simulink model "bh_3d_pend_sim_compare"  (R2017a)
settings: Solver=ode45  StartTime=0.0  StopTime=11  RelTol=1e-5  EnableMultiTasking=on
undefined symbols (not defined in the file or in its folder): DOT_Phi_Theta_Psi, DOT_XYZ, g, Hx, Hy, Hz, Lx, Ly, Lz, M_cart, m_pend, Phi_Theta_Psi, q0_ang_deg, q0_dot_and_deg, X, XYZ, Y, Z
libraries: nesl_utility x14, sm_lib x9, simulink_extras x5
settings Model: Creator=bhorton  LastModifiedBy=bhorton
settings SolverCC: ZeroCrossAlgorithm=Adaptive
settings DataIOCC: LimitDataPoints=on
settings OptimizationCC: LifeSpan=inf
settings DebuggingCC: AllowSymbolicDim=off  SFUnexpectedBacktrackingDiag=warning  SFNoUnconditionalDefaultTransitionDiag=warning  SFExecutionAtInitializationDiag=none
settings GRTTargetCC: TargetLangStandard=C89/C90 (ANSI)  GeneratePreprocessorConditionals=Disable all
settings ConfigComp: CovMetricSettings=dw  CovHtmlReporting=on  CovSaveCumulativeToWorkspaceVar=on  CovSaveSingleToWorkspaceVar=on  CovExternalEMLEnable=off  CovSFcnEnable=off
settings SimscapeCC: SimscapeLogType=all  SimscapeLogDataHistory=10000
settings ConfigurationSet: Description=SimMechanics 2G

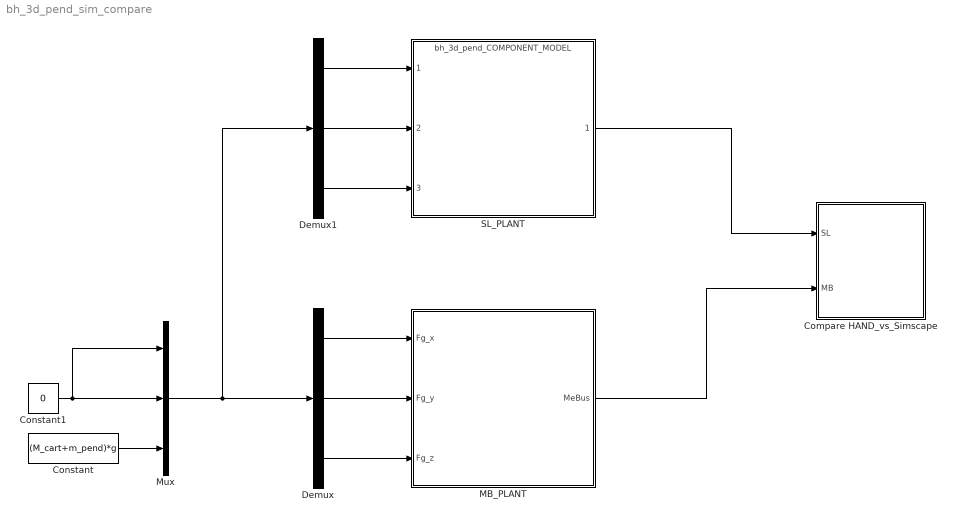
== system bh_3d_pend_sim_compare ==
  Compare HAND_vs_Simscape : Subsystem
  Constant : Constant  Value=(M_cart+m_pend)*g
  Constant1 : Constant  Value=0
  Demux : Demux  Outputs=3
  Demux1 : Demux  Outputs=3
  MB_PLANT : Subsystem
  Mux : Mux  Inputs=3
  SL_PLANT : ModelReference  ModelNameDialog=bh_3d_pend_COMPONENT_MODEL.slx  SimulationMode=Normal  ModelReferenceVersion=1.15
  wires:
  Constant/1 -> Mux/3
  Constant1/1 -> Mux/1, Mux/2
  Demux/1 -> MB_PLANT/1(Fg_x)
  Demux/3 -> MB_PLANT/3(Fg_z)
  Demux/2 -> MB_PLANT/2(Fg_y)
  Mux/1 -> Demux1/1, Demux/1
  Demux1/1 -> SL_PLANT/1
  Demux1/2 -> SL_PLANT/2
  Demux1/3 -> SL_PLANT/3
  SL_PLANT/1 -> Compare HAND_vs_Simscape/1(SL)
  MB_PLANT/1(MeBus) -> Compare HAND_vs_Simscape/2(MB)

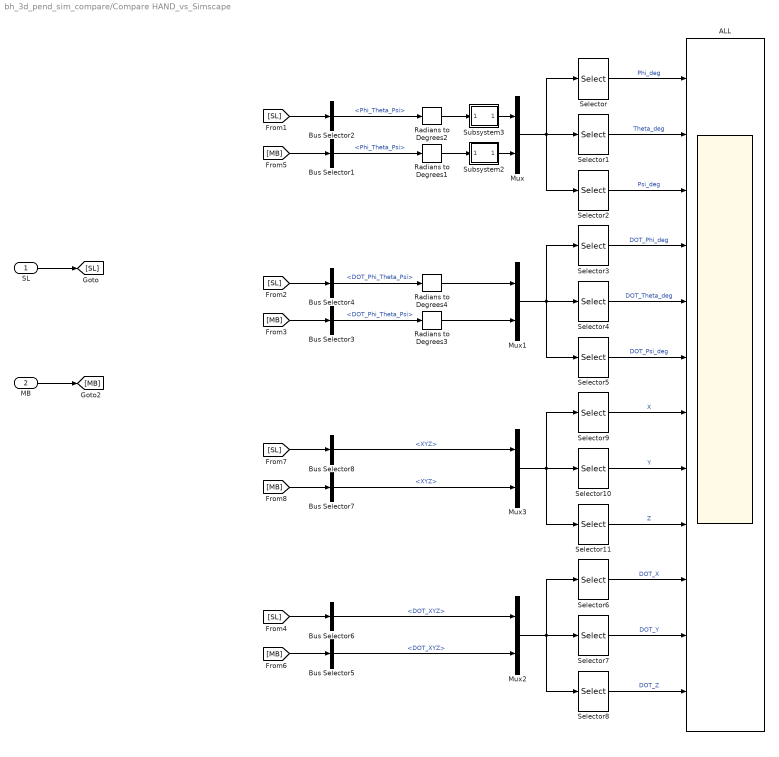
== system bh_3d_pend_sim_compare/Compare HAND_vs_Simscape ==
  SL : Inport
  MB : Inport  Port=2
  ALL : Scope  NumInputPorts=12
  Bus Selector1 : BusSelector  OutputSignals=Phi_Theta_Psi
  Bus Selector2 : BusSelector  OutputSignals=Phi_Theta_Psi
  Bus Selector3 : BusSelector  OutputSignals=DOT_Phi_Theta_Psi
  Bus Selector4 : BusSelector  OutputSignals=DOT_Phi_Theta_Psi
  Bus Selector5 : BusSelector  OutputSignals=DOT_XYZ
  Bus Selector6 : BusSelector  OutputSignals=DOT_XYZ
  Bus Selector7 : BusSelector  OutputSignals=XYZ
  Bus Selector8 : BusSelector  OutputSignals=XYZ
  Mux{,1..3} (4 alike) : Mux  Inputs=2
  Radians to Degrees{1..4} (4 alike) : simulink_extras/Transformations/Radians to Degrees
  Selector{,3,6,9} (4 alike) : Selector  InputPortWidth=6  IndexOptions=Index vector (dialog)  Indices=[1 4]  OutputSizes=1
  Selector{1,4,7,10} (4 alike) : Selector  InputPortWidth=6  IndexOptions=Index vector (dialog)  Indices=[2 5]  OutputSizes=1
  Selector{2,5,8,11} (4 alike) : Selector  InputPortWidth=6  IndexOptions=Index vector (dialog)  Indices=[3 6]  OutputSizes=1
  Subsystem2 : Subsystem
      mask Display: disp(sprintf('Mod\n360'))
  Subsystem3 : Subsystem
      mask Display: disp(sprintf('Mod\n360'))
  wires:
  SL/1 -> [SL]
  MB/1 -> [MB]
  [MB] -> Bus Selector1/1
  Bus Selector1/1 -> Radians to Degrees1/1  "<Phi_Theta_Psi>"
  [SL] -> Bus Selector2/1
  Bus Selector2/1 -> Radians to Degrees2/1  "<Phi_Theta_Psi>"
  Radians to Degrees2/1 -> Subsystem3/1(In1)
  Subsystem2/1(Out1) -> Mux/2
  Subsystem3/1(Out1) -> Mux/1
  Radians to Degrees1/1 -> Subsystem2/1(In1)
  Selector/1 -> ALL/1  "Phi_deg"
  Selector2/1 -> ALL/3  "Psi_deg"
  Selector1/1 -> ALL/2  "Theta_deg"
  Mux/1 -> Selector2/1, Selector/1, Selector1/1
  [MB] -> Bus Selector3/1
  Bus Selector3/1 -> Radians to Degrees3/1  "<DOT_Phi_Theta_Psi>"
  Radians to Degrees3/1 -> Mux1/2
  [SL] -> Bus Selector4/1
  Bus Selector4/1 -> Radians to Degrees4/1  "<DOT_Phi_Theta_Psi>"
  Radians to Degrees4/1 -> Mux1/1
  Mux1/1 -> Selector5/1, Selector3/1, Selector4/1
  Selector4/1 -> ALL/5  "DOT_Theta_deg"
  Selector3/1 -> ALL/4  "DOT_Phi_deg"
  Selector5/1 -> ALL/6  "DOT_Psi_deg"
  Mux2/1 -> Selector8/1, Selector6/1, Selector7/1
  Bus Selector6/1 -> Mux2/1  "<DOT_XYZ>"
  [SL] -> Bus Selector6/1
  Bus Selector5/1 -> Mux2/2  "<DOT_XYZ>"
  [MB] -> Bus Selector5/1
  Selector7/1 -> ALL/11  "DOT_Y"
  Selector8/1 -> ALL/12  "DOT_Z"
  Selector6/1 -> ALL/10  "DOT_X"
  [MB] -> Bus Selector7/1
  Bus Selector7/1 -> Mux3/2  "<XYZ>"
  [SL] -> Bus Selector8/1
  Bus Selector8/1 -> Mux3/1  "<XYZ>"
  Mux3/1 -> Selector11/1, Selector9/1, Selector10/1
  Selector9/1 -> ALL/7  "X"
  Selector10/1 -> ALL/8  "Y"
  Selector11/1 -> ALL/9  "Z"

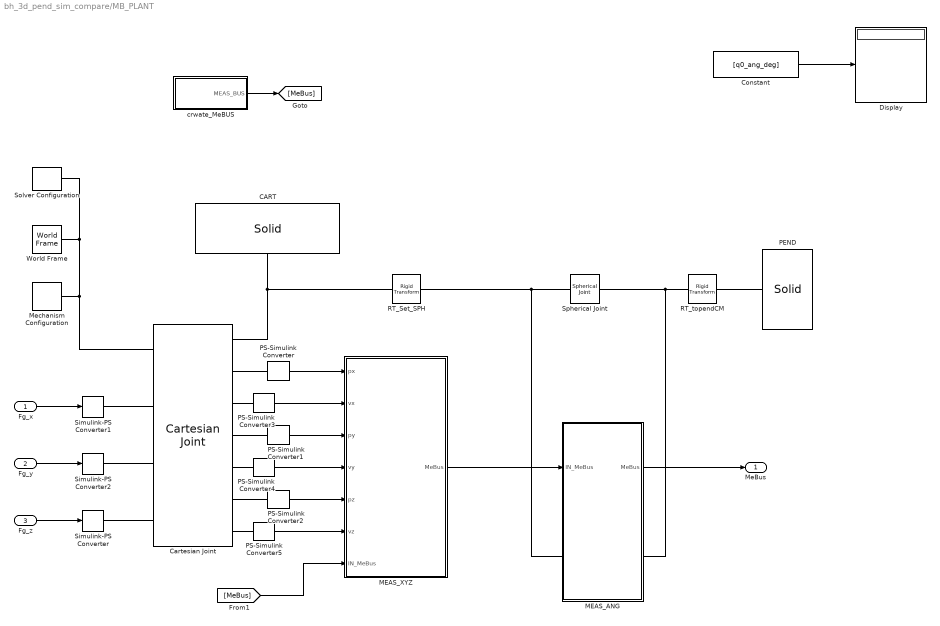
== system bh_3d_pend_sim_compare/MB_PLANT ==
  Fg_x : Inport
  Fg_y : Inport  Port=2
  Fg_z : Inport  Port=3
  CART : sm_lib/Body Elements/Solid  InertiaType=PointMass  Mass=M_cart  MassUnits=kg  CenterOfMass=[0 0 0]  CenterOfMassUnits=m  MomentsOfInertia=[1 1 1]  MomentsOfInertiaUnits=kg*m^2  ProductsOfInertia=[0 0 0]  ProductsOfInertiaUnits=kg*m^2  DensityBased=off  Density=1000  DensityUnits=kg/(m^3)  DoExposeReferenceFrame=on  SerializedFrames=<Frames/>  GraphicType=FromGeometry  MarkerShape=Sphere  MarkerSize=10  MarkerSizeUnits=m  GraphicVisPropType=SimpleVisualProperties  GraphicDiffuseColor=[0.2 0.2 1.0]  GraphicSpecularColor=[0.5 0.5 0.5 1.0]  GraphicAmbientColor=[0.15 0.15 0.15 1.0]  GraphicEmissiveColor=[0.0 0.0 0.0 1.0]  GraphicShininess=75  GraphicOpacity=1.0  GeometryShape=Brick  RectangleSize=[1 1]  RectangleSizeUnits=m  BrickDimensions=[Hx, Hy, Hz]  BrickDimensionUnits=m  CylinderRadius=1  CylinderRadiusUnits=m  CylinderLength=1  CylinderLengthUnits=m  SphereRadius=1  SphereRadiusUnits=m  EllipsoidRadii=[1 1 1]  EllipsoidRadiiUnits=m  ExtrusionCrossSection=[1 1; -1 1; -1 -1; 1 -1]  ExtrusionCrossSectionUnits=m  ExtrusionLength=1  ExtrusionLengthUnits=m  PolygonNumSides=3  PolygonOuterRadius=1  PolygonOuterRadiusUnits=m  ExtGeomFileType=STL  ExtGeomFileUnits=m  RevolutionCrossSection=[1 1; 1 -1; 2 -1; 2 1]  RevolutionCrossSectionUnits=m  RevolutionExtent=Full  RevolutionAngle=180  RevolutionAngleUnits=deg
  Cartesian Joint : sm_lib/Joints/Cartesian Joint  SenseConstraintForce=off  SenseConstraintForceX=off  SenseConstraintForceY=off  SenseConstraintForceZ=off  SenseConstraintTorque=off  SenseConstraintTorqueX=off  SenseConstraintTorqueY=off  SenseConstraintTorqueZ=off  SenseTotalForce=off  SenseTotalForceX=off  SenseTotalForceY=off  SenseTotalForceZ=off  SenseTotalTorque=off  SenseTotalTorqueX=off  SenseTotalTorqueY=off  SenseTotalTorqueZ=off  CompositeWrenchDir=FollowerOnBase  CompositeWrenchFrame=BaseFrame  PxEquilibriumPosition=0  PxEquilibriumPositionUnits=m  PxSpringStiffness=0  PxSpringStiffnessUnits=N/m  PxDampingCoefficient=0  PxDampingCoefficientUnits=N/(m/s)  PxTorqueActuationMode=InputTorque  PxMotionActuationMode=ComputedMotion  PxSensePosition=on  PxSenseVelocity=on  PxSenseAcceleration=off  PxSenseTorqueForce=off  PxPositionTargetSpecify=off  PxPositionTargetPriority=High  PxPositionTargetValue=0  PxPositionTargetValueUnits=m  PxVelocityTargetSpecify=off  PxVelocityTargetPriority=High  PxVelocityTargetValue=0  PxVelocityTargetValueUnits=m/s  PyEquilibriumPosition=0  PyEquilibriumPositionUnits=m  PySpringStiffness=0  PySpringStiffnessUnits=N/m  PyDampingCoefficient=0  PyDampingCoefficientUnits=N/(m/s)  PyTorqueActuationMode=InputTorque  PyMotionActuationMode=ComputedMotion  PySensePosition=on  PySenseVelocity=on  PySenseAcceleration=off  PySenseTorqueForce=off  PyPositionTargetSpecify=off  PyPositionTargetPriority=High  PyPositionTargetValue=0  PyPositionTargetValueUnits=m  PyVelocityTargetSpecify=off  PyVelocityTargetPriority=High  PyVelocityTargetValue=0  PyVelocityTargetValueUnits=m/s  PzEquilibriumPosition=0  PzEquilibriumPositionUnits=m  PzSpringStiffness=0  PzSpringStiffnessUnits=N/m  PzDampingCoefficient=0  PzDampingCoefficientUnits=N/(m/s)  PzTorqueActuationMode=InputTorque  PzMotionActuationMode=ComputedMotion  PzSensePosition=on  PzSenseVelocity=on  PzSenseAcceleration=off  PzSenseTorqueForce=off  PzPositionTargetSpecify=off  PzPositionTargetPriority=High  PzPositionTargetValue=0  PzPositionTargetValueUnits=m  PzVelocityTargetSpecify=off  PzVelocityTargetPriority=High  PzVelocityTargetValue=0  PzVelocityTargetValueUnits=m/s
  Constant : Constant  Value=[q0_ang_deg]  VectorParams1D=off
  Display : Display
  MEAS_ANG : Subsystem
  MEAS_XYZ : Subsystem
  Mechanism Configuration : sm_lib/Utilities/Mechanism Configuration  UniformGravity=Constant  GravityVector=[0 0 -9.80665]  GravityUnits=m/s^2  LinearizationDelta=0.001
  PEND : sm_lib/Body Elements/Solid  InertiaType=CalculateFromGeometry  Mass=m_pend  MassUnits=kg  CenterOfMass=[0 0 0]  CenterOfMassUnits=m  MomentsOfInertia=[1 1 1]  MomentsOfInertiaUnits=kg*m^2  ProductsOfInertia=[0 0 0]  ProductsOfInertiaUnits=kg*m^2  DensityBased=off  Density=1000  DensityUnits=kg/(m^3)  DoExposeReferenceFrame=on  SerializedFrames=<Frames/>  GraphicType=FromGeometry  MarkerShape=Sphere  MarkerSize=10  MarkerSizeUnits=m  GraphicVisPropType=SimpleVisualProperties  GraphicDiffuseColor=[1.0 0.6 0.2]  GraphicSpecularColor=[0.5 0.5 0.5 1.0]  GraphicAmbientColor=[0.15 0.15 0.15 1.0]  GraphicEmissiveColor=[0.0 0.0 0.0 1.0]  GraphicShininess=75  GraphicOpacity=1.0  GeometryShape=Brick  RectangleSize=[1 1]  RectangleSizeUnits=m  BrickDimensions=[Lx, Ly, Lz]  BrickDimensionUnits=m  CylinderRadius=1  CylinderRadiusUnits=m  CylinderLength=1  CylinderLengthUnits=m  SphereRadius=1  SphereRadiusUnits=m  EllipsoidRadii=[1 1 1]  EllipsoidRadiiUnits=m  ExtrusionCrossSection=[1 1; -1 1; -1 -1; 1 -1]  ExtrusionCrossSectionUnits=m  ExtrusionLength=1  ExtrusionLengthUnits=m  PolygonNumSides=3  PolygonOuterRadius=1  PolygonOuterRadiusUnits=m  ExtGeomFileType=STL  ExtGeomFileUnits=m  RevolutionCrossSection=[1 1; 1 -1; 2 -1; 2 1]  RevolutionCrossSectionUnits=m  RevolutionExtent=Full  RevolutionAngle=180  RevolutionAngleUnits=deg
  PS-Simulink Converter : nesl_utility/PS-Simulink Converter  PhysicalDomain=network_engine_domain  SubClassName=ps_output  LeftPortType=input  RightPortType=output  PseudoPeriodic=off  Frequencies=[]  Unit=m  AffineConversion=off
  PS-Simulink Converter1 : nesl_utility/PS-Simulink Converter  PhysicalDomain=network_engine_domain  SubClassName=ps_output  LeftPortType=input  RightPortType=output  PseudoPeriodic=off  Frequencies=[]  Unit=m  AffineConversion=off
  PS-Simulink Converter2 : nesl_utility/PS-Simulink Converter  PhysicalDomain=network_engine_domain  SubClassName=ps_output  LeftPortType=input  RightPortType=output  PseudoPeriodic=off  Frequencies=[]  Unit=m  AffineConversion=off
  PS-Simulink Converter3 : nesl_utility/PS-Simulink Converter  PhysicalDomain=network_engine_domain  SubClassName=ps_output  LeftPortType=input  RightPortType=output  PseudoPeriodic=off  Frequencies=[]  Unit=m/s  AffineConversion=off
  PS-Simulink Converter4 : nesl_utility/PS-Simulink Converter  PhysicalDomain=network_engine_domain  SubClassName=ps_output  LeftPortType=input  RightPortType=output  PseudoPeriodic=off  Frequencies=[]  Unit=m/s  AffineConversion=off
  PS-Simulink Converter5 : nesl_utility/PS-Simulink Converter  PhysicalDomain=network_engine_domain  SubClassName=ps_output  LeftPortType=input  RightPortType=output  PseudoPeriodic=off  Frequencies=[]  Unit=m/s  AffineConversion=off
  RT_Set_SPH : sm_lib/Frames and Transforms/Rigid Transform  TranslationMethod=StandardAxis  TranslationStandardOffset=Tv_Z  TranslationLengthUnit=m  TranslationStandardAxis=+Z  TranslationCartesianOffset=[0 0 0]  TranslationROffset=0  TranslationROffsetUnits=m  TranslationZOffset=0  TranslationZOffsetUnits=m  TranslationThetaOffset=0  TranslationThetaOffsetUnits=deg  RotationMethod=None  RotationAngleUnits=deg  RotationStandardAxis=+Z  RotationAngle=0  RotationArbitraryAxis=[0 0 1]  FollAlignAxisA=+X  BaseAlignAxisA=+Y  FollAlignAxisB=+Y  BaseAlignAxisB=+Z  RotationSequenceAxes=FollowerAxes  RotationSequence=XYX  RotationSequenceAngles=[0 0 0]  RotationSequenceAnglesUnits=deg  RotationMatrix=[1 0 0; 0 1 0; 0 0 1]
  RT_topendCM : sm_lib/Frames and Transforms/Rigid Transform  TranslationMethod=StandardAxis  TranslationStandardOffset=Lz/2  TranslationLengthUnit=m  TranslationStandardAxis=+Z  TranslationCartesianOffset=[0 0 0]  TranslationROffset=0  TranslationROffsetUnits=m  TranslationZOffset=0  TranslationZOffsetUnits=m  TranslationThetaOffset=0  TranslationThetaOffsetUnits=deg  RotationMethod=None  RotationAngleUnits=deg  RotationStandardAxis=+Z  RotationAngle=0  RotationArbitraryAxis=[0 0 1]  FollAlignAxisA=+X  BaseAlignAxisA=+Y  FollAlignAxisB=+Y  BaseAlignAxisB=+Z  RotationSequenceAxes=FollowerAxes  RotationSequence=XYX  RotationSequenceAngles=[0 0 0]  RotationSequenceAnglesUnits=deg  RotationMatrix=[1 0 0; 0 1 0; 0 0 1]
  Simulink-PS Converter : nesl_utility/Simulink-PS Converter  PhysicalDomain=network_engine_domain  SubClassName=ps_input  LeftPortType=input  RightPortType=output  PseudoPeriodic=off  Frequencies=[]  NoiseDistribution=none  NoiseParameters=[]  Unit=N  AffineConversion=off  FilteringAndDerivatives=zero  SimscapeFilterOrder=1  InputFilterTimeConstant=0.001  UdotUserProvided=1
  Simulink-PS Converter1 : nesl_utility/Simulink-PS Converter  PhysicalDomain=network_engine_domain  SubClassName=ps_input  LeftPortType=input  RightPortType=output  PseudoPeriodic=off  Frequencies=[]  NoiseDistribution=none  NoiseParameters=[]  Unit=N  AffineConversion=off  FilteringAndDerivatives=zero  SimscapeFilterOrder=1  InputFilterTimeConstant=0.001  UdotUserProvided=1
  Simulink-PS Converter2 : nesl_utility/Simulink-PS Converter  PhysicalDomain=network_engine_domain  SubClassName=ps_input  LeftPortType=input  RightPortType=output  PseudoPeriodic=off  Frequencies=[]  NoiseDistribution=none  NoiseParameters=[]  Unit=N  AffineConversion=off  FilteringAndDerivatives=zero  SimscapeFilterOrder=1  InputFilterTimeConstant=0.001  UdotUserProvided=1
  Solver Configuration : nesl_utility/Solver Configuration  PhysicalDomain=network_engine_domain  SubClassName=solver  LeftPortType=input  RightPortType=generic  Accelerate=off  Tones=[]  Harmonics=[]  SimulateNoise=off  Profile=off  UseLocalSampling=off  EnableSwitchedLinearOptims=on  FrequencyDomain=off  UseCCode=off  RelTol=0.001  AbsTol=1e-06  MinStep=1e-09  ToWorkspace=off  RevertToSquareIcSolve=off  NumHomotopyIterations=100  PhasorMode=off  PhasorModeNumHarmonics=1  OverrideAbsTol=off  DoDC=off  ResidualTolerance=1e-09  UseLocalSolver=off  LocalSolverChoice=NE_BACKWARD_EULER_ADVANCER  LocalSolverSampleTime=0.001  DoFixedCost=off  MaxNonlinIter=3  MaxModeIter=2  LinearAlgebra=Sparse  DelaysMemoryBudget=1024  AutomaticFiltering=on  FilteringTimeConstant=0.001
  Spherical Joint : sm_lib/Joints/Spherical Joint  SenseConstraintForce=off  SenseConstraintForceX=off  SenseConstraintForceY=off  SenseConstraintForceZ=off  SenseConstraintTorque=off  SenseConstraintTorqueX=off  SenseConstraintTorqueY=off  SenseConstraintTorqueZ=off  SenseTotalForce=off  SenseTotalForceX=off  SenseTotalForceY=off  SenseTotalForceZ=off  SenseTotalTorque=off  SenseTotalTorqueX=off  SenseTotalTorqueY=off  SenseTotalTorqueZ=off  CompositeWrenchDir=FollowerOnBase  CompositeWrenchFrame=BaseFrame  DefPosRotationMethod=None  DefPosRotationAngleUnits=deg  DefPosRotationStandardAxis=+Z  DefPosRotationAngle=0.0  DefPosRotationArbitraryAxis=[0 0 1]  DefPosFollAlignAxisA=+X  DefPosBaseAlignAxisA=+Y  DefPosFollAlignAxisB=+Y  DefPosBaseAlignAxisB=+Z  DefPosRotationSequenceAxes=FollowerAxes  DefPosRotationSequence=XYX  DefPosRotationSequenceAngles=[0 0 0]  DefPosRotationSequenceAnglesUnits=deg  DefPosRotationMatrix=[1 0 0; 0 1 0; 0 0 1]  EqPosRotationMethod=None  EqPosRotationAngleUnits=deg  EqPosRotationStandardAxis=+Z  EqPosRotationAngle=0.0  EqPosRotationArbitraryAxis=[0 0 1]  EqPosFollAlignAxisA=+X  EqPosBaseAlignAxisA=+Y  EqPosFollAlignAxisB=+Y  EqPosBaseAlignAxisB=+Z  EqPosRotationSequenceAxes=FollowerAxes  EqPosRotationSequence=XYX  EqPosRotationSequenceAngles=[0 0 0]  EqPosRotationSequenceAnglesUnits=deg  EqPosRotationMatrix=[1 0 0; 0 1 0; 0 0 1]  SpringStiffness=0  SpringStiffnessUnits=N*m/deg  DampingCoefficient=0  DampingCoefficientUnits=N*m/(deg/s)  ActuateTorqueX=off  ActuateTorqueY=off  ActuateTorqueZ=off  ActuateTorque=off  TorqueActuationMode=NoTorque  MotionActuationMode=ComputedMotion  ActuationFrame=BaseFrame  SensePosition=off  SenseVelocityX=off  SenseVelocityY=off  SenseVelocityZ=off  SenseVelocity=off  SenseAccelerationX=off  SenseAccelerationY=off  SenseAccelerationZ=off  SenseAcceleration=off  SenseTorqueX=off  SenseTorqueY=off  SenseTorqueZ=off  SenseTorqueForce=off  SensingFrame=BaseFrame  PositionTargetRotationMethod=RotationSequence  PositionTargetRotationAngleUnits=deg  PositionTargetRotationStandardAxis=+Z  PositionTargetRotationAngle=0.0  PositionTargetRotationArbitraryAxis=[0 0 1]  PositionTargetFollAlignAxisA=+X  PositionTargetBaseAlignAxisA=+Y  PositionTargetFollAlignAxisB=+Y  PositionTargetBaseAlignAxisB=+Z  PositionTargetRotationSequenceAxes=FollowerAxes  PositionTargetRotationSequence=ZYX  PositionTargetRotationSequenceAngles=[q0_ang_deg]  PositionTargetRotationSequenceAnglesUnits=deg  PositionTargetRotationMatrix=[1 0 0; 0 1 0; 0 0 1]  PositionTargetSpecify=on  PositionTargetPriority=High  VelocityTargetValue=[q0_dot_and_deg]  VelocityTargetValueUnits=deg/s  VelocityTargetSpecify=on  VelocityTargetPriority=High  VelocityTargetInFollowerFrame=on
      settings: AttributesFormatString=|
      | %<PositionTargetRotationSequenceAnglesUnits>
      | %<PositionTargetRotationSequenceAngles>
      | %<PositionTargetRotationSequence>
  World Frame : sm_lib/Frames and Transforms/World Frame
  crwate_MeBUS : Subsystem
  MeBus : Outport
  wires:
  Fg_z/1 -> Simulink-PS Converter/1
  Fg_y/1 -> Simulink-PS Converter2/1
  Fg_x/1 -> Simulink-PS Converter1/1
  crwate_MeBUS/1(MEAS_BUS) -> [MeBus]
  MEAS_XYZ/1(MeBus) -> MEAS_ANG/1(IN_MeBus)
  PS-Simulink Converter2/1 -> MEAS_XYZ/5(pz)
  PS-Simulink Converter1/1 -> MEAS_XYZ/3(py)
  PS-Simulink Converter3/1 -> MEAS_XYZ/2(vx)
  PS-Simulink Converter/1 -> MEAS_XYZ/1(px)
  PS-Simulink Converter4/1 -> MEAS_XYZ/4(vy)
  PS-Simulink Converter5/1 -> MEAS_XYZ/6(vz)
  [MeBus] -> MEAS_XYZ/7(IN_MeBus)
  MEAS_ANG/1(MeBus) -> MeBus/1
  Constant/1 -> Display/1
  connections:
  Spherical Joint/LConn1 -- MEAS_ANG/LConn1 -- RT_Set_SPH/RConn1
  Mechanism Configuration/RConn1 -- Solver Configuration/RConn1 -- World Frame/RConn1 -- Cartesian Joint/LConn1
  RT_topendCM/LConn1 -- MEAS_ANG/RConn1 -- Spherical Joint/RConn1
  CART/RConn1 -- Cartesian Joint/RConn1 -- RT_Set_SPH/LConn1
  RT_topendCM/RConn1 -- PEND/RConn1
  Simulink-PS Converter/RConn1 -- Cartesian Joint/LConn4
  Simulink-PS Converter2/RConn1 -- Cartesian Joint/LConn3
  Simulink-PS Converter1/RConn1 -- Cartesian Joint/LConn2
  PS-Simulink Converter2/LConn1 -- Cartesian Joint/RConn6
  Cartesian Joint/RConn4 -- PS-Simulink Converter1/LConn1
  Cartesian Joint/RConn2 -- PS-Simulink Converter/LConn1
  Cartesian Joint/RConn7 -- PS-Simulink Converter5/LConn1
  Cartesian Joint/RConn5 -- PS-Simulink Converter4/LConn1
  Cartesian Joint/RConn3 -- PS-Simulink Converter3/LConn1

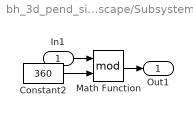
== system bh_3d_pend_sim_compare/Compare HAND_vs_Simscape/Subsystem2 ==
  In1 : Inport
  Constant2 : Constant  Value=360
  Math Function : Math  Operator=mod  SaturateOnIntegerOverflow=on
  Out1 : Outport
  wires:
  Math Function/1 -> Out1/1
  In1/1 -> Math Function/1
  Constant2/1 -> Math Function/2

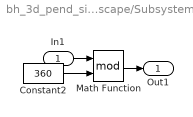
== system bh_3d_pend_sim_compare/Compare HAND_vs_Simscape/Subsystem3 ==
  In1 : Inport
  Constant2 : Constant  Value=360
  Math Function : Math  Operator=mod  SaturateOnIntegerOverflow=on
  Out1 : Outport
  wires:
  Math Function/1 -> Out1/1
  In1/1 -> Math Function/1
  Constant2/1 -> Math Function/2

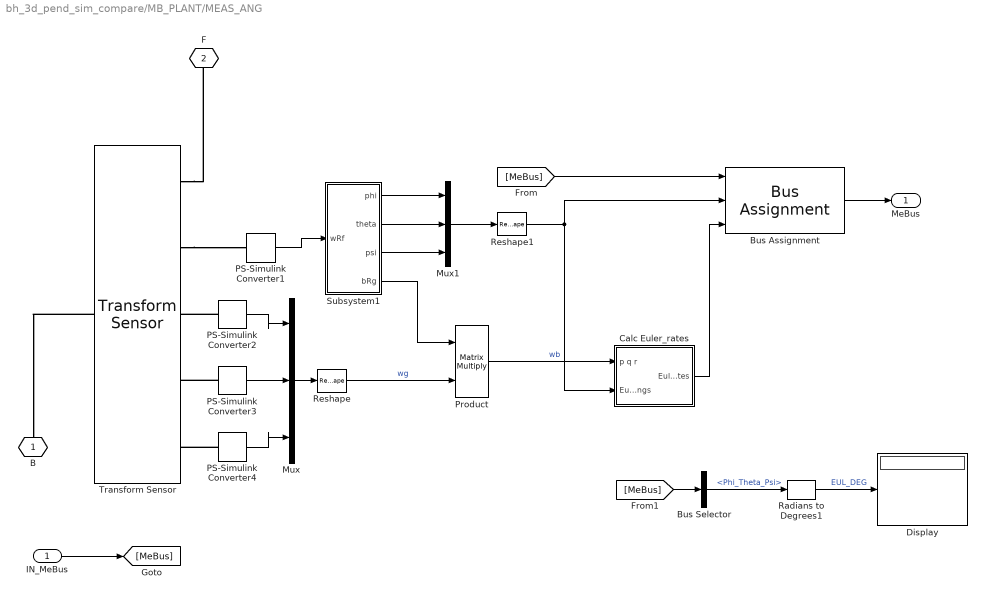
== system bh_3d_pend_sim_compare/MB_PLANT/MEAS_ANG ==
  IN_MeBus : Inport
  Bus Assignment : BusAssignment  AssignedSignals=Phi_Theta_Psi,DOT_Phi_Theta_Psi
  Bus Selector : BusSelector  OutputSignals=Phi_Theta_Psi
  Calc Euler_rates : Subsystem
  Display : Display
  Mux : Mux  Inputs=3
  Mux1 : Mux  Inputs=3
  PS-Simulink Converter1 : nesl_utility/PS-Simulink Converter  PhysicalDomain=network_engine_domain  SubClassName=ps_output  LeftPortType=input  RightPortType=output  PseudoPeriodic=off  Frequencies=[]  Unit=1  AffineConversion=off
  PS-Simulink Converter2 : nesl_utility/PS-Simulink Converter  PhysicalDomain=network_engine_domain  SubClassName=ps_output  LeftPortType=input  RightPortType=output  PseudoPeriodic=off  Frequencies=[]  Unit=rad/s  AffineConversion=off
  PS-Simulink Converter3 : nesl_utility/PS-Simulink Converter  PhysicalDomain=network_engine_domain  SubClassName=ps_output  LeftPortType=input  RightPortType=output  PseudoPeriodic=off  Frequencies=[]  Unit=rad/s  AffineConversion=off
  PS-Simulink Converter4 : nesl_utility/PS-Simulink Converter  PhysicalDomain=network_engine_domain  SubClassName=ps_output  LeftPortType=input  RightPortType=output  PseudoPeriodic=off  Frequencies=[]  Unit=rad/s  AffineConversion=off
  Product : Product  Multiplication=Matrix(*)
  Radians to Degrees1 : simulink_extras/Transformations/Radians to Degrees
  Reshape : Reshape  OutputDimensionality=Column vector (2-D)
  Reshape1 : Reshape  OutputDimensionality=Column vector (2-D)
  Subsystem1 : Subsystem
  Transform Sensor : sm_lib/Frames and Transforms/Transform Sensor  MeasurementFrame=World  SenseAngle=off  SenseAxis=off  SenseAngle1=off  SenseAngle2=off  SenseAngle3=off  SenseQ=off  SenseR=on  SenseOmegaX=on  SenseOmegaY=on  SenseOmegaZ=on  SenseOmega1=off  SenseOmega2=off  SenseOmega3=off  SenseQDot=off  SenseRDot=off  SenseAlphaX=off  SenseAlphaY=off  SenseAlphaZ=off  SenseAlpha1=off  SenseAlpha2=off  SenseAlpha3=off  SenseQDDot=off  SenseRDDot=off  SenseX=off  SenseY=off  SenseZ=off  SenseRad=off  SenseAzim=off  SenseDist=off  SenseInc=off  SenseXDot=off  SenseYDot=off  SenseZDot=off  SenseRadDot=off  SenseAzimDot=off  SenseDistDot=off  SenseIncDot=off  SenseXDDot=off  SenseYDDot=off  SenseZDDot=off  SenseRadDDot=off  SenseAzimDDot=off  SenseDistDDot=off  SenseIncDDot=off
  B : PMIOPort  Port=1  Side=Left
  F : PMIOPort  Port=2  Side=Right
  MeBus : Outport
  wires:
  PS-Simulink Converter1/1 -> Subsystem1/1(wRf)
  Subsystem1/1(phi) -> Mux1/1
  Subsystem1/3(psi) -> Mux1/3
  PS-Simulink Converter2/1 -> Mux/1
  PS-Simulink Converter3/1 -> Mux/2
  PS-Simulink Converter4/1 -> Mux/3
  Mux/1 -> Reshape/1
  Subsystem1/4(bRg) -> Product/1
  Reshape/1 -> Product/2  "wg"
  Product/1 -> Calc Euler_rates/1("p q r ")  "wb"
  Subsystem1/2(theta) -> Mux1/2
  IN_MeBus/1 -> [MeBus]
  Mux1/1 -> Reshape1/1
  [MeBus] -> Bus Assignment/1
  Reshape1/1 -> Bus Assignment/2, Calc Euler_rates/2(Euler_angs)
  Calc Euler_rates/1(Euler_rates) -> Bus Assignment/3
  Bus Assignment/1 -> MeBus/1
  [MeBus] -> Bus Selector/1
  Bus Selector/1 -> Radians to Degrees1/1  "<Phi_Theta_Psi>"
  Radians to Degrees1/1 -> Display/1  "EUL_DEG"
  connections:
  PS-Simulink Converter2/LConn1 -- Transform Sensor/RConn3
  PS-Simulink Converter4/LConn1 -- Transform Sensor/RConn5
  PS-Simulink Converter3/LConn1 -- Transform Sensor/RConn4
  Transform Sensor/LConn1 -- B/RConn1
  Transform Sensor/RConn1 -- F/RConn1
  Transform Sensor/RConn2 -- PS-Simulink Converter1/LConn1

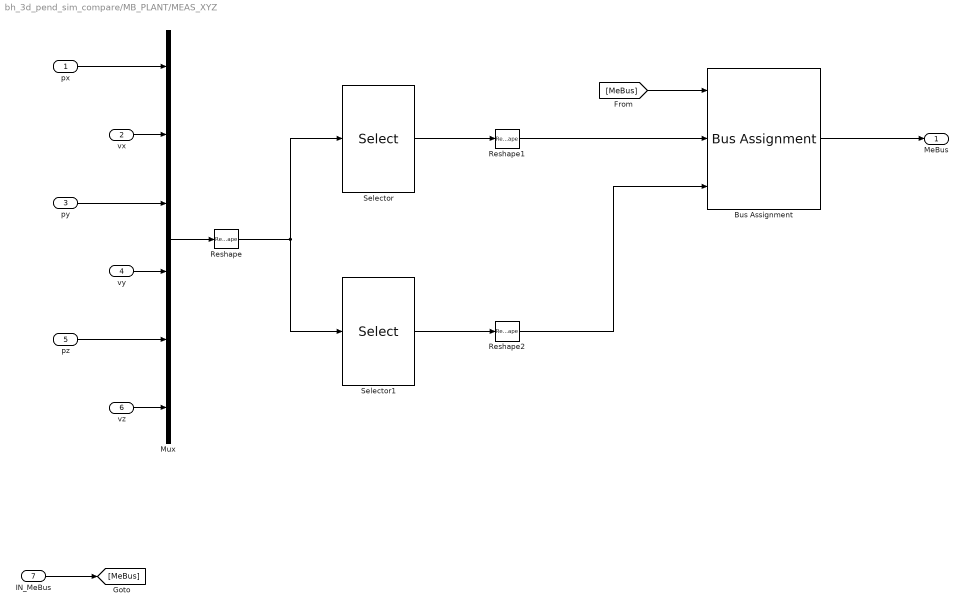
== system bh_3d_pend_sim_compare/MB_PLANT/MEAS_XYZ ==
  px : Inport
  vx : Inport  Port=2
  py : Inport  Port=3
  vy : Inport  Port=4
  pz : Inport  Port=5
  vz : Inport  Port=6
  IN_MeBus : Inport  Port=7
  Bus Assignment : BusAssignment  AssignedSignals=XYZ,DOT_XYZ
  Mux : Mux  Inputs=6
  Reshape : Reshape  OutputDimensionality=Column vector (2-D)
  Reshape1 : Reshape  OutputDimensionality=Column vector (2-D)
  Reshape2 : Reshape  OutputDimensionality=Column vector (2-D)
  Selector : Selector  InputPortWidth=6  IndexOptions=Index vector (dialog)  Indices=[1 3 5]  OutputSizes=1
  Selector1 : Selector  InputPortWidth=6  IndexOptions=Index vector (dialog)  Indices=[2 4 6]  OutputSizes=1
  MeBus : Outport
  wires:
  vz/1 -> Mux/6
  pz/1 -> Mux/5
  vy/1 -> Mux/4
  py/1 -> Mux/3
  vx/1 -> Mux/2
  px/1 -> Mux/1
  Mux/1 -> Reshape/1
  Reshape/1 -> Selector1/1, Selector/1
  Selector/1 -> Reshape1/1
  Selector1/1 -> Reshape2/1
  IN_MeBus/1 -> [MeBus]
  [MeBus] -> Bus Assignment/1
  Bus Assignment/1 -> MeBus/1
  Reshape1/1 -> Bus Assignment/2
  Reshape2/1 -> Bus Assignment/3

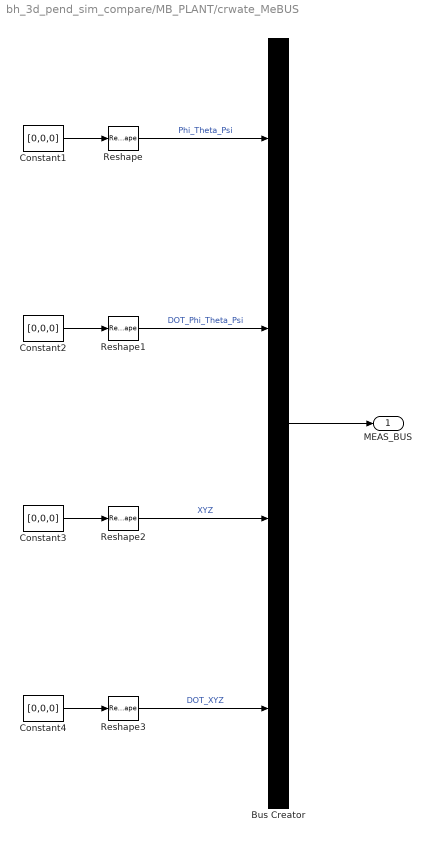
== system bh_3d_pend_sim_compare/MB_PLANT/crwate_MeBUS ==
  Bus Creator : BusCreator  Inputs=4
  Constant{1..4} (4 alike) : Constant  Value=[0,0,0]
  Reshape{,1..3} (4 alike) : Reshape  OutputDimensionality=Column vector (2-D)
  MEAS_BUS : Outport
  wires:
  Reshape/1 -> Bus Creator/1  "Phi_Theta_Psi"
  Reshape1/1 -> Bus Creator/2  "DOT_Phi_Theta_Psi"
  Reshape2/1 -> Bus Creator/3  "XYZ"
  Reshape3/1 -> Bus Creator/4  "DOT_XYZ"
  Constant1/1 -> Reshape/1
  Constant2/1 -> Reshape1/1
  Constant3/1 -> Reshape2/1
  Constant4/1 -> Reshape3/1
  Bus Creator/1 -> MEAS_BUS/1

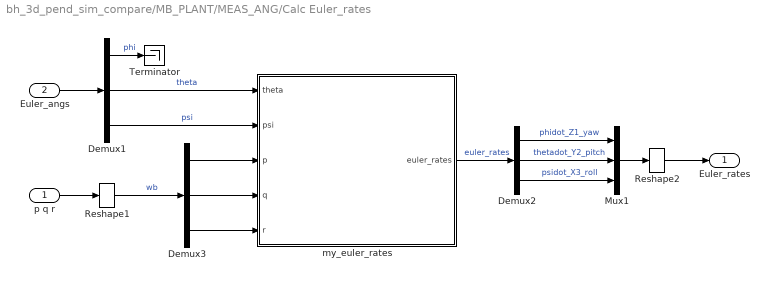
== system bh_3d_pend_sim_compare/MB_PLANT/MEAS_ANG/Calc Euler_rates ==
  "p q r " : Inport
  Euler_angs : Inport  Port=2
  Demux1 : Demux  Outputs=3
  Demux2 : Demux  Outputs=3
  Demux3 : Demux  Outputs=3
  Mux1 : Mux  Inputs=3
  Reshape1 : Reshape  OutputDimensionality=Column vector (2-D)
  Reshape2 : Reshape  OutputDimensionality=Column vector (2-D)
  Terminator : Terminator
  my_euler_rates : MATLAB Function  TreatAsAtomicUnit=on
  Euler_rates : Outport
  wires:
  Reshape1/1 -> Demux3/1  "wb"
  my_euler_rates/1(euler_rates) -> Demux2/1  "euler_rates"
  Demux2/3 -> Mux1/3  "psidot_X3_roll"
  Demux2/2 -> Mux1/2  "thetadot_Y2_pitch"
  Demux2/1 -> Mux1/1  "phidot_Z1_yaw"
  Reshape2/1 -> Euler_rates/1
  Mux1/1 -> Reshape2/1
  Demux3/3 -> my_euler_rates/5(r)
  Demux3/2 -> my_euler_rates/4(q)
  Demux3/1 -> my_euler_rates/3(p)
  Euler_angs/1 -> Demux1/1
  "p q r "/1 -> Reshape1/1
  Demux1/2 -> my_euler_rates/1(theta)  "theta"
  Demux1/1 -> Terminator/1  "phi"
  Demux1/3 -> my_euler_rates/2(psi)  "psi"

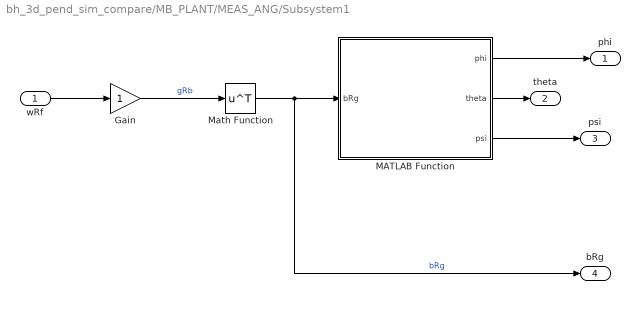
== system bh_3d_pend_sim_compare/MB_PLANT/MEAS_ANG/Subsystem1 ==
  wRf : Inport
  Gain : Gain
  MATLAB Function : MATLAB Function  TreatAsAtomicUnit=on
  Math Function : Math  Operator=transpose  SaturateOnIntegerOverflow=on
  phi : Outport
  theta : Outport  Port=2
  psi : Outport  Port=3
  bRg : Outport  Port=4
  wires:
  wRf/1 -> Gain/1
  Gain/1 -> Math Function/1  "gRb"
  Math Function/1 -> bRg/1, MATLAB Function/1(bRg)  "bRg"
  MATLAB Function/1(phi) -> phi/1
  MATLAB Function/2(theta) -> theta/1
  MATLAB Function/3(psi) -> psi/1

== matlab function bh_3d_pend_sim_compare/MB_PLANT/MEAS_ANG/Subsystem1/MATLAB Function ==
  data: bRg input; phi output; theta output; psi output
function [phi, theta, psi] = calc_EUL(bRg)
%#codegen

% bRg = [ ...
%                               cos(phi)*cos(theta),                              cos(theta)*sin(phi),         -sin(theta);
%  cos(phi)*sin(psi)*sin(theta) - cos(psi)*sin(phi), cos(phi)*cos(psi) + sin(phi)*sin(psi)*sin(theta), cos(theta)*sin(psi);
%  sin(phi)*sin(psi) + cos(phi)*cos(psi)*sin(theta), cos(psi)*sin(phi)*sin(theta) - cos(phi)*sin(psi), cos(psi)*cos(theta);
%  ];

phi   = 0; 
theta = 0;
psi   = 0;

theta = -asin(  bRg(1,3) ); % so +/- pi/2 range

phi   = atan2( bRg(1,2) , bRg(1,1)  );  % so +/- pi range
psi   = atan2( bRg(2,3) , bRg(3,3)  );  % so +/- pi range


% THE_TAN_PHI =  bRg(1,2) / bRg(1,1);
% 
% phi   = atan2( THE_TAN_PHI  );  % so +/- pi range
% 
% THE_TAN_PSI =  bRg(2,3) / bRg(3,3);
% 
% psi   = atan2( THE_TAN_PSI  );  % so +/- pi range


% convert to [0 2pi]
% if(phi < 0)   
%     phi = pi + (pi - abs(phi) );   
% end
% 
% if(psi < 0)   
%     psi = pi + (pi - abs(psi) );   
% end

end %function

== matlab function bh_3d_pend_sim_compare/MB_PLANT/MEAS_ANG/Calc Euler_rates/my_euler_rates ==
  data: theta input; euler_rates output; psi input; p input; q input; r input
function euler_rates = my_euler_rates(theta,psi,p,q,r)
%#codegen

%    This function was generated by the Symbolic Math Toolbox version 7.0.
%    09-Jun-2016 10:28:25

euler_rates = [(r.*cos(psi)+q.*sin(psi))./cos(theta);
                q.*cos(psi)-r.*sin(psi);
               (p.*cos(theta)+r.*cos(psi).*sin(theta)+q.*sin(psi).*sin(theta))./cos(theta)];
